simulink model "mdl1"  (Simulink 8.1)
settings: Solver=ode1  StartTime=0.0  StopTime=5  FixedStep=0.01  RelTol=1e-3
libraries: simulink_need_slupdate x1
settings Model: Creator=adasubu  LastModifiedBy=adasubu  ExtModeArmWhenConnect=off  BufferReuse=off
settings DataIOCC: SignalLoggingName=sigsOut
settings OptimizationCC: BlockReduction=off  ConditionallyExecuteInputs=off  OptimizeBlockIOStorage=off  BufferReuse=off  ExpressionFolding=off  ExpressionDepthLimit=128  LocalBlockOutputs=off
settings DebuggingCC: SaveWithParameterizedLinksMsg=none  SignalResolutionControl=TryResolveAllWithWarning  SolverPrmCheckMsg=none  MultiTaskDSMMsg=warning  MultiTaskCondExecSysMsg=none  FcnCallInpInsideContextMsg=EnableAllAsError  StrictBusMsg=None
settings HardwareCC: TargetUnknown=on
settings RTWCC: SystemTargetFile=rti1102.tlc  MakeCommand=make_rti  TemplateMakefile=rti1102.tmf  RetainRTWFile=on  ProcessScript=rti1102_make_rtw_hook  IncludeERTFirstTime=on
settings STFCustomTargetCC: CodeReplacementLibrary=ANSI_C  ModelReferenceCompliant=off  GeneratePreprocessorConditionals=Disable all  MATLABClassNameForMDSCustomization=Simulink.SoftwareTarget.TargetSpecificTriggerConfigurationBase  SystemTargetFile=rti1102.tlc

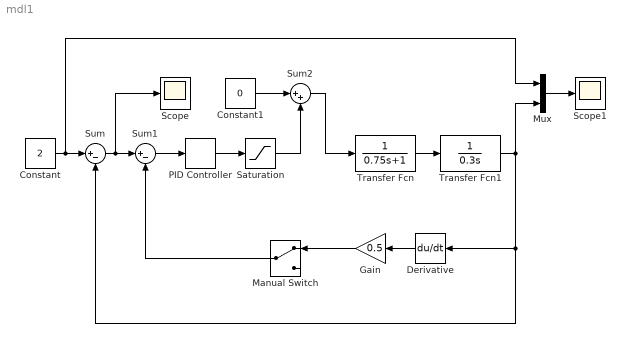
== system mdl1 ==
  Constant : Constant  Value=2
  Constant1 : Constant  Value=0
  Derivative : Derivative
  Gain : Gain  Gain=0.5  SaturateOnIntegerOverflow=on  OutDataTypeStr=Inherit: Same as input  ParamDataTypeStr=Inherit: Same as input
  Manual Switch : ManualSwitch
  Mux : Mux  Inputs=2
  PID Controller : simulink_need_slupdate/PID Controller  P=50  I=1  D=10
  Saturation : Saturate  UpperLimit=5  LowerLimit=-5
  Scope : Scope
  Scope1 : Scope
      settings: TimeRange=5
  Sum : Sum  Inputs=|+-  SaturateOnIntegerOverflow=on
  Sum1 : Sum  Inputs=|+-  SaturateOnIntegerOverflow=on
  Sum2 : Sum  Inputs=|++  SaturateOnIntegerOverflow=on
  Transfer Fcn : TransferFcn  Denominator=[0.75 1]
  Transfer Fcn1 : TransferFcn  Denominator=[0.3 0]
  wires:
  Constant/1 -> Sum/1, Mux/1
  Sum/1 -> Sum1/1, Scope/1
  Sum1/1 -> PID Controller/1
  PID Controller/1 -> Saturation/1
  Saturation/1 -> Sum2/2
  Constant1/1 -> Sum2/1
  Transfer Fcn/1 -> Transfer Fcn1/1
  Sum2/1 -> Transfer Fcn/1
  Transfer Fcn1/1 -> Mux/2, Derivative/1, Sum/2
  Derivative/1 -> Gain/1
  Gain/1 -> Manual Switch/1
  Manual Switch/1 -> Sum1/2
  Mux/1 -> Scope1/1
